simulink model "mass_ramp"  (R2023a)
settings: Solver=VariableStepAuto  StartTime=0.0  StopTime=10.0  RelTol=1e-3
undefined symbols (not defined in the file): b, F, g, k, m, phi, x0, x_dot0
settings Model: Creator=m260477  LastModifiedBy=m260477
settings DataIOCC: Refine=10

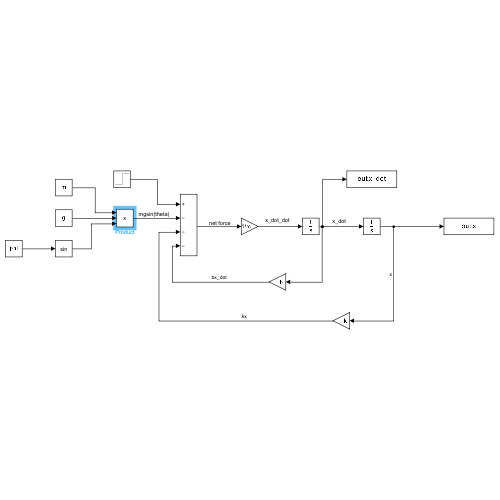
[thumbnail: Simulink's stored preview of the top-level diagram]
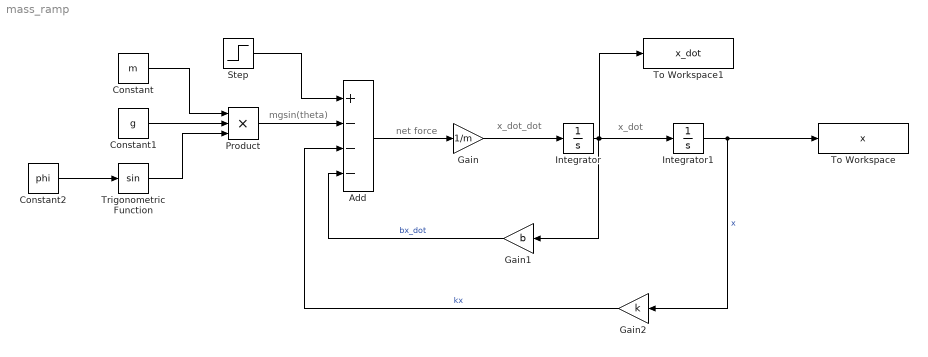
== system mass_ramp ==
  note: mgsin(theta)
  note: net force
  note: x_dot
  note: x_dot_dot
  Add : Sum  Inputs=+---
  Constant : Constant  Value=m
  Constant1 : Constant  Value=g
  Constant2 : Constant  Value=phi
  Gain : Gain  Gain=1/m
  Gain1 : Gain  Gain=b
  Gain2 : Gain  Gain=k
  Integrator : Integrator  InitialCondition=x_dot0
  Integrator1 : Integrator  InitialCondition=x0
  Product : Product  Inputs=3  RndMeth=Zero
  Step : Step  Time=0  After=F  SampleTime=0
  To Workspace : ToWorkspace  VariableName=x  SaveFormat=Timeseries  SampleTime=-1
  To Workspace1 : ToWorkspace  VariableName=x_dot  SaveFormat=Timeseries  SampleTime=-1
  Trigonometric Function : Trigonometry
  wires:
  Add/1 -> Gain/1
  Gain/1 -> Integrator/1
  Integrator/1 -> Gain1/1, To Workspace1/1, Integrator1/1
  Gain1/1 -> Add/4  "bx_dot"
  Integrator1/1 -> To Workspace/1, Gain2/1  "x"
  Gain2/1 -> Add/3  "kx"
  Constant2/1 -> Trigonometric Function/1
  Constant1/1 -> Product/2
  Trigonometric Function/1 -> Product/3
  Constant/1 -> Product/1
  Product/1 -> Add/2
  Step/1 -> Add/1
